simulink model "Test3C25Board"  (Simulink 6.3)
settings: Solver=ode45  SolverMode=SingleTasking  StartTime=0.0  StopTime=100.0  FixedStep=1  RelTol=1e-3
InitFcn:
  | %% DSPBuilder Start
  | alt_dspbuilder_update_model(bdroot)
  | %% DSPBuilder End
libraries: Cyclone_III_EP3C25_alteradspbuilder2 x9, allblocks_alteradspbuilder2 x6
settings Model: LastModifiedBy=LKONG  StrictBusMsg=None
settings DataIOCC: SignalLoggingName=sigsOut
settings OptimizationCC: InlineInvariantSignals=on
settings DebuggingCC: SolverPrmCheckMsg=none
settings HardwareCC: TargetUnknown=on
settings GRTTargetCC: ModelReferenceCompliant=off  MatFileLogging=off

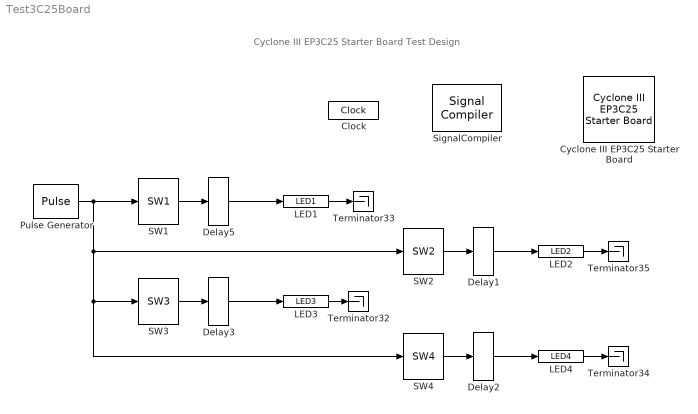
== system Test3C25Board ==
  note: Cyclone III EP3C25 Starter Board Test Design
  Clock : allblocks_alteradspbuilder2/Clock  ClockPeriod=10  ClockPeriodUnit=ns  SampleTime=1  SimulationStartCycle=5  PhaseOffset=0  Reset=aclr  ResetType=Active Low  Export=off
  Cyclone III EP3C25 Starter Board : Cyclone_III_EP3C25_alteradspbuilder2/Cyclone III EP3C25 Starter Board  ClockPinIn=Pin_B9  GlobalResetPin=Pin_N2  device=EP3C25F324C8
  Delay{1..3,5} (4 alike) : allblocks_alteradspbuilder2/Delay  pipeline=1  ClockPhase=1  use_ena=off  use_sclr=off  use_init=off  reset_value=1
  LED1 : Cyclone_III_EP3C25_alteradspbuilder2/LED1  iofile=D:\ws72\workspace\Documentation\DesignExamples\Demos\Board\CycloneIII_DSPBoard_3C25\tb_Test3C25Board\Test3C25Board_LED1.capture  externalType=Inferred  location=Pin_P13
  LED2 : Cyclone_III_EP3C25_alteradspbuilder2/LED2  iofile=D:\ws72\workspace\Documentation\DesignExamples\Demos\Board\CycloneIII_DSPBoard_3C25\tb_Test3C25Board\Test3C25Board_LED2.capture  externalType=Inferred  location=Pin_P12
  LED3 : Cyclone_III_EP3C25_alteradspbuilder2/LED3  iofile=D:\ws72\workspace\Documentation\DesignExamples\Demos\Board\CycloneIII_DSPBoard_3C25\tb_Test3C25Board\Test3C25Board_LED3.capture  externalType=Inferred  location=Pin_N12
  LED4 : Cyclone_III_EP3C25_alteradspbuilder2/LED4  iofile=D:\ws72\workspace\Documentation\DesignExamples\Demos\Board\CycloneIII_DSPBoard_3C25\tb_Test3C25Board\Test3C25Board_LED4.capture  externalType=Inferred  location=Pin_N9
  Pulse Generator : DiscretePulseGenerator  Period=20000  PulseWidth=2
  SW1 : Cyclone_III_EP3C25_alteradspbuilder2/SW1  iofile=D:\ws72\workspace\Documentation\DesignExamples\Demos\Board\CycloneIII_DSPBoard_3C25\tb_Test3C25Board\Test3C25Board_SW1.salt  externalType=Inferred  SpecifyClock=off  location=Pin_F1
  SW2 : Cyclone_III_EP3C25_alteradspbuilder2/SW2  iofile=D:\ws72\workspace\Documentation\DesignExamples\Demos\Board\CycloneIII_DSPBoard_3C25\tb_Test3C25Board\Test3C25Board_SW2.salt  externalType=Inferred  SpecifyClock=off  location=Pin_F2
  SW3 : Cyclone_III_EP3C25_alteradspbuilder2/SW3  iofile=D:\ws72\workspace\Documentation\DesignExamples\Demos\Board\CycloneIII_DSPBoard_3C25\tb_Test3C25Board\Test3C25Board_SW3.salt  externalType=Inferred  SpecifyClock=off  location=Pin_A10
  SW4 : Cyclone_III_EP3C25_alteradspbuilder2/SW4  iofile=D:\ws72\workspace\Documentation\DesignExamples\Demos\Board\CycloneIII_DSPBoard_3C25\tb_Test3C25Board\Test3C25Board_SW4.salt  externalType=Inferred  SpecifyClock=off  location=Pin_B10
  SignalCompiler : allblocks_alteradspbuilder2/Signal Compiler  DeviceFamily=Cyclone III  DeviceName=EP3C25F324C8  EnableSignalTap=on  SignalTapDepth=512  UseBoardBlock=on  StpUseDefaultClock=on  StpClock=Clock
  Terminator{32..35} (4 alike) : Terminator
  wires:
  SW1/1 -> Delay5/1
  SW2/1 -> Delay1/1
  SW3/1 -> Delay3/1
  SW4/1 -> Delay2/1
  Delay2/1 -> LED4/1
  Delay3/1 -> LED3/1
  Delay1/1 -> LED2/1
  Delay5/1 -> LED1/1
  LED3/1 -> Terminator32/1
  LED1/1 -> Terminator33/1
  LED4/1 -> Terminator34/1
  LED2/1 -> Terminator35/1
  Pulse Generator/1 -> SW3/1, SW4/1, SW2/1, SW1/1
